simulink model "model_main5"  (R2023b)
settings: Solver=ode4  StartTime=0.0  StopTime=1000  FixedStep=dt  RelTol=1e-3
InitFcn:
  | model_init
values from neighbouring files (symbols this model uses):
  dt = 0.01    [model_init.m]
  Iws = diag([1 1 1 1])*0.2274    [model_init.m]
  m_tot = 3300    [model_init.m]
  norm_Ib = diag(diag(SC_Ib) / norm(diag(SC_Ib)))    [model_init.m]
  Omega1_init = 2000*rpm2rad    (= 209.439510239)    [model_init.m]
  Omega2_init = 2000*rpm2rad    (= 209.439510239)    [model_init.m]
  Omega3_init = 2000*rpm2rad    (= 209.439510239)    [model_init.m]
  Omega4_init = 2000*rpm2rad    (= 209.439510239)    [model_init.m]
  Omega_ref = [1000 1000 1000 1000]*rpm2rad    [model_init.m]
  port_offset = [7.196; 0 ; 0.618]    [model_init.m]
  qb0 = angle2quat(ag0(1),ag0(2),ag0(3),'ZYX')'    [model_init.m]
  rad2rpm = 1/rpm2rad    (= 9.54929658551)    [model_init.m]
  RCS_F = 1.0    (= 1)    [model_init.m]
  RCS_Pos = [RCS1_POS , RCS2_POS , RCS3_POS , RCS4_POS ,            RCS5_POS , RCS6_POS , RCS7_POS , RCS8_POS ,            RCS9_POS , RCS10_POS, RCS11_POS, RCS12_POS,            RCS13_POS, RCS14_POS, RCS15_POS, RCS16_POS]    [model_init.m]
  RCS_PWM_Freq = 0.1    [model_init.m]
  RCS_Sampling_time = 0.01    [model_init.m]
  RCS_THR_vec = [RCS1_THR , RCS2_THR , RCS3_THR , RCS4_THR,                 RCS5_THR , RCS6_THR , RCS7_THR , RCS8_THR,                 RCS9_THR , RCS10_THR, RCS11_THR, RCS12_THR,                 RCS13_THR, RCS14_THR, RCS15_THR, RCS16_THR]    [model_init.m]
  REL_port_POS_I_0 = REL_TS_POS_I_0 - quat2rotm(qb0') * port_offset    [model_init.m]
  REL_port_VEL_I_0 = REL_TS_VEL_I_0 - quat2rotm(qb0') * cross(wb0,port_offset)    [model_init.m]
  REL_TS_POS_I_0 = TS_pos0 - SC_pos0    [model_init.m]
  REL_TS_VEL_I_0 = TS_vel0 - SC_vel0    [model_init.m]
  RW_As = [RW1_Axis,RW2_Axis,RW3_Axis,RW4_Axis]    [model_init.m]
  RW_Max_Speed = 4200*rpm2rad    (= 439.822971503)    [model_init.m]
  RW_t_max = 0.5    [model_init.m]
  SC_Ib = [1843.56  -0.0019  -803.89 ... (first row only)    [model_init.m]
  SC_state0 = kepel_statvec (SC_Kepler)    [model_init.m]
  TS_Ib = diag([1 1 1])    [model_init.m]
  TS_qb0 = angle2quat(deg2rad(0),deg2rad(0),deg2rad(0),'ZYX')'    [model_init.m]
  TS_state0 = kepel_statvec (TS_Kepler)    [model_init.m]
  TS_wb0 = deg2rad([0 0 0]')    [model_init.m]
  wb0 = deg2rad([-0.3 -0.1 0.2])'    [model_init.m]
undefined symbols (not defined in the file or in its folder): RCS_F_vec, RCS_pos, SS_Total_Mass, TC_Kepler
libraries: simulink x16, simulink_extras x16, aerolibutil x9, sharedtransform x8
(part 3 of 3)

== matlab function model_main5/Enabled Subsystem/QP Controller2 ==
  settings: updateMethod=DISCRETE
  data: RCS_F_cmd output; RCS_tau_cmd output; F_pd_in input; tau_pd_in input; u_rw_cmd output; tau_rw_body output; tau_dump_ref output; Omega_rw_in input; Omega_ref_in input; RW_max_speed input; F_rcs_max_in input; tau_rcs_max_in input; k_dump input; eta_rw input; eta_tau_rcs input; eta_F input; v_tau input; v_dump input; v_F input; dt input; s_tau output; s_dump output; s_F output; exitflag_out output
function [RCS_F_cmd, RCS_tau_cmd, u_rw_cmd, tau_rw_body, tau_dump_ref, s_tau, s_dump, s_F, exitflag_out] = ...
    QP_CA_RW_RCS_WRENCH(F_pd_in, tau_pd_in, Omega_rw_in, Omega_ref_in, ...
    RW_max_speed, F_rcs_max_in, tau_rcs_max_in, ...
    k_dump, eta_rw, eta_tau_rcs, eta_F,  v_tau, v_dump, v_F, dt)

% Wrench-level QP control allocation
% - RW  : actuator-level (4 wheel torques)
% - RCS : wrench-level (3-axis force + 3-axis torque)
%
% Decision variable:
% z = [u_rw(4); tau_rcs(3); F_rcs(3); s_tau(3); s_dump(3); s_F(3)] -> 19
%
% Equality constraints:
%   -As*u_rw + tau_rcs - s_tau   = tau_pd
%    tau_rcs       - s_dump      = tau_dump_ref
%    F_rcs         - s_F         = F_pd
%
% Inputs
%   F_pd_in        [3x1] desired body force from position PD [N]
%   tau_pd_in      [3x1] desired body torque from attitude PD [N*m]
%   Omega_rw_in    [4x1] current wheel speeds [rad/s]
%   Omega_ref_in   [4x1] desired wheel speeds [rad/s]
%   RW_max_speed   [1x1] wheel speed limit [rad/s]
%   F_rcs_max_in   [3x1] approximate RCS body force bounds [N]
%   tau_rcs_max_in [3x1] approximate RCS body torque bounds [N*m]
%   k_dump         [1x1] momentum dumping gain [1/s]
%   eta_rw         [1x1] RW effort weight
%   eta_F          [1x1] RCS force effort weight
%   eta_rcs        [1x1] RCS torque effort weight
%   v_tau          [1x1] attitude slack weight
%   v_dump         [1x1] dumping slack weight
%   v_F            [1x1] force slack weight
%   dt             [1x1] sample time [s]
%
% Outputs
%   RCS_F_cmd      [3x1] body force command to existing RCS allocator [N]
%   RCS_tau_cmd    [3x1] body torque command to existing RCS allocator [N*m]
%   u_rw_cmd       [4x1] wheel torque command [N*m]
%   tau_rw_body    [3x1] RW-generated body torque [N*m]
%   tau_dump_ref   [3x1] desired dumping torque reference [N*m]
%   s_tau          [3x1] attitude torque slack
%   s_dump         [3x1] dumping torque slack
%   s_F            [3x1] force slack
%   exitflag_out   [1x1] quadprog exitflag

persistent z_save

if isempty(z_save)
    z_save = zeros(19,1);
end

%% outputs
RCS_F_cmd    = zeros(3,1);
RCS_tau_cmd  = zeros(3,1);
u_rw_cmd     = zeros(4,1);
tau_rw_body  = zeros(3,1);
tau_dump_ref = zeros(3,1);
s_tau        = zeros(3,1);
s_dump       = zeros(3,1);
s_F          = zeros(3,1);
exitflag_out = 0;

% for i = 1:3
%     if F_pd_in(i) >= F_rcs_max_in(i)
%         F_pd_in(i) = F_rcs_max_in(i);
%     elseif F_pd_in(i) <= -F_rcs_max_in(i)
%         F_pd_in(i) = -F_rcs_max_in(i);
%     end
% end
% 

%% fixed-size local copies
F_pd = zeros(3,1);
F_pd(1) = F_pd_in(1);
F_pd(2) = F_pd_in(2);
F_pd(3) = F_pd_in(3);

tau_pd = zeros(3,1);
tau_pd(1) = tau_pd_in(1);
tau_pd(2) = tau_pd_in(2);
tau_pd(3) = tau_pd_in(3);

Omega_rw = zeros(4,1);
Omega_rw(1) = Omega_rw_in(1);
Omega_rw(2) = Omega_rw_in(2);
Omega_rw(3) = Omega_rw_in(3);
Omega_rw(4) = Omega_rw_in(4);

Omega_ref = zeros(4,1);
Omega_ref(1) = Omega_ref_in(1);
Omega_ref(2) = Omega_ref_in(2);
Omega_ref(3) = Omega_ref_in(3);
Omega_ref(4) = Omega_ref_in(4);

F_rcs_max = zeros(3,1);
F_rcs_max(1) = abs(F_rcs_max_in(1));
F_rcs_max(2) = abs(F_rcs_max_in(2));
F_rcs_max(3) = abs(F_rcs_max_in(3));

tau_rcs_max = zeros(3,1);
tau_rcs_max(1) = abs(tau_rcs_max_in(1));
tau_rcs_max(2) = abs(tau_rcs_max_in(2));
tau_rcs_max(3) = abs(tau_rcs_max_in(3));

if dt <= 1e-6
    dt = 1e-6;
end

if RW_max_speed <= 1e-6
    RW_max_speed = 1e-6;
end

%% RW geometry
% tau_rw_body = -As * u_rw
As = [ 0.70710678,  0.0,        -0.70710678,  0.0;
    0.0,         0.70710678,  0.0,        -0.70710678;
    0.70710678,  0.70710678,  0.70710678,  0.70710678 ];

% wheel spin inertias [kg*m^2]
Jw = 0.2274 * ones(4,1);

%% actuator limits
% RW torque limits
u_rw_max = 0.5 * ones(4,1)  ;
u_rw_min = -u_rw_max;

% RW torque-rate limits
du_max = 20.0 * ones(4,1);   % [N*m/s]
du_min = -du_max;

% RW speed limits
Omega_max = RW_max_speed * ones(4,1) - 10;
Omega_min = -Omega_max;

%% previous solution
z_prev = z_save;
u_prev = z_prev(1:4);

%% virtual momentum dumping torque
% tau_dump_ref = -k_dump * h_rw_err
% h_rw_err = As * diag(Jw) * (Omega_rw - Omega_ref)
omega_err = Omega_rw - Omega_ref;
h_rw_err  = As * (Jw .* omega_err);   % [N*m*s]
tau_dump_ref = -k_dump * h_rw_err;    % [N*m]

%% QP cost
% z = [u_rw(4); tau_rcs(3); F_rcs(3); s_tau(3); s_dump(3); s_F(3)]
H = zeros(19,19);
f = zeros(19,1);

% effort weights
H = 2*diag([eta_rw*ones(4,1); ...
    eta_tau_rcs*ones(3,1); ...
    eta_F*ones(3,1); ...
    v_tau*ones(3,1); ...
    v_dump*ones(3,1); ...
    v_F*ones(3,1);]);
%%%%%%%%%%%%%
u_rw_scale   = u_rw_max;               % [N*m]
tau_scale    = tau_rcs_max(:);         % [N*m]
F_scale      = F_rcs_max(:);           % [N]

s_tau_scale  = tau_rcs_max(:) + abs(As)*u_rw_max;           % [N*m]
s_dump_scale = tau_rcs_max(:);           % [N*m]
s_F_scale    = F_rcs_max(:);             % [N]

scale_vec = [u_rw_scale;
             tau_scale; 
             F_scale;
             s_tau_scale;
             s_dump_scale;
             s_F_scale];

weight_vec = [eta_rw      * ones(4,1);
              eta_tau_rcs * ones(3,1);
              eta_F       * ones(3,1);
              v_tau       * ones(3,1);
              v_dump      * ones(3,1);
              v_F         * ones(3,1)];

H = 2 * diag(weight_vec ./ (scale_vec.^2  ));
%%%%%%%%%%%%%
% optional small RW smoothing
wr = 1e-3;
H(1,1) = H(1,1) + 2*wr;
H(2,2) = H(2,2) + 2*wr;
H(3,3) = H(3,3) + 2*wr;
H(4,4) = H(4,4) + 2*wr;
f(1:4) = -2*wr*u_prev;

% numerical symmetry
H = 0.5*(H + H') + 1e-9*eye(19);

%% equality constraints
% -As*u_rw + tau_rcs - s_tau  = tau_pd
%  tau_rcs       - s_dump     = tau_dump_ref
%  F_rcs         - s_F        = F_pd

Aeq = [       -As, eye(3), zeros(3,3),    -eye(3), zeros(3,3), zeros(3,3);
    zeros(3,4), eye(3), zeros(3,3), zeros(3,3),    -eye(3), zeros(3,3);
    zeros(3,4), zeros(3,3), eye(3), zeros(3,3), zeros(3,3),   -eye(3)];

beq = [tau_pd;
    tau_dump_ref;
    F_pd];

%% bounds
% RW torque-rate bounds
lb_rate = u_prev + du_min * dt;
ub_rate = u_prev + du_max * dt;

% RW speed-next bounds
% Omega_next = Omega_rw + dt*(u_rw./Jw)
lb_speed = Jw .* ((Omega_min - Omega_rw) / dt);
ub_speed = Jw .* ((Omega_max - Omega_rw) / dt);

% final RW bounds
lb_u = max(u_rw_min, max(lb_rate, lb_speed));
ub_u = min(u_rw_max, min(ub_rate, ub_speed));


% feasibility repair
for i = 1:4
    if lb_u(i) > ub_u(i)
        c = 0.5 * (lb_u(i) + ub_u(i));
        lb_u(i) = c;
        ub_u(i) = c;
    end
end

% RCS force bounds
lb_F = -F_rcs_max;
ub_F =  F_rcs_max;

% RCS torque bounds
lb_t = -tau_rcs_max;
ub_t =  tau_rcs_max;

% slack bounds
big = 1e6;
lb_s_tau  = -big * ones(3,1);
ub_s_tau  =  big * ones(3,1);
lb_s_dump = -big * ones(3,1);
ub_s_dump =  big * ones(3,1);
lb_s_F    = -big * ones(3,1);
ub_s_F    =  big * ones(3,1);

lb = [lb_u; lb_t; lb_F; lb_s_tau; lb_s_dump; lb_s_F];
ub = [ub_u; ub_t; ub_F; ub_s_tau; ub_s_dump; ub_s_F];

%% initial guess (make it equality-feasible)
u0 = min(max(u_prev, lb_u), ub_u);

F0 = F_pd;
for i = 1:3
    if F0(i) > ub_F(i)
        F0(i) = ub_F(i);
    elseif F0(i) < lb_F(i)
        F0(i) = lb_F(i);
    end
end

t0 = tau_dump_ref;
for i = 1:3
    if t0(i) > ub_t(i)
        t0(i) = ub_t(i);
    elseif t0(i) < lb_t(i)
        t0(i) = lb_t(i);
    end
end

s_tau0  = -As*u0 + t0 - tau_pd;
s_dump0 = t0 - tau_dump_ref;
s_F0    = F0 - F_pd;

x0 = [u0;
    t0;
    F0;
    s_tau0;
    s_dump0;
    s_F0];

%% solve
A = zeros(0,19);
b = zeros(0,1);

options = optimoptions('quadprog', ...
    'Algorithm', 'active-set', ...
    'Display', 'off', ...
    'ConstraintTolerance', 1e-6, ...
    'OptimalityTolerance', 1e-6, ...
    'StepTolerance', 1e-12, ...
    'MaxIterations', 60);

[z, ~, exitflag] = quadprog(H, f, A, b, Aeq, beq, lb, ub, x0, options);

if isempty(z) || exitflag <= 0
    z = x0;
end

%% outputs
u_rw_cmd    = z(1:4);
RCS_tau_cmd = z(5:7);
RCS_F_cmd   = z(8:10);

s_tau  = z(11:13);
s_dump = z(14:16);
s_F    = z(17:19);

tau_rw_body = -As * u_rw_cmd;

z_save = z;
exitflag_out = exitflag;
end

== matlab function model_main5/probe1 ==
  data: TS_p_I input; rel_port_pos output; SS_p_I input; TS_v_I input; SS_v_I input; q input; wb input; port_offset input; rel_port_vel output
function [rel_port_pos, rel_port_vel] = fcn(TS_p_I, SS_p_I, TS_v_I, SS_v_I, q, wb, port_offset) 
% port_offset : chaser CG-docking port offset    [7.196; 0 ; 0.618]
% q : body to eci
 
 
port_pos_I = SS_p_I + quat_to_dcm_sf(q) * port_offset;
port_vel_I = SS_v_I + quat_to_dcm_sf(q) * cross(wb,port_offset);

% Relative position based on docking ports

rel_port_pos = TS_p_I - port_pos_I;
rel_port_vel = TS_v_I - port_vel_I;
 
end

function C = quat_to_dcm_sf(q)
% scalar-first quaternion, body -> reference   quat2rotm
q = q / (sqrt(sum(q.^2)) + 1e-12);

qw = q(1);
qx = q(2);
qy = q(3);
qz = q(4);

C = [1-2*(qy*qy+qz*qz),   2*(qx*qy-qw*qz),   2*(qx*qz+qw*qy);
    2*(qx*qy+qw*qz),     1-2*(qx*qx+qz*qz), 2*(qy*qz-qw*qx);
    2*(qx*qz-qw*qy),     2*(qy*qz+qw*qx),   1-2*(qx*qx+qy*qy)];
end

== matlab function model_main5/Enabled Subsystem/QP Controller1 ==
  settings: updateMethod=DISCRETE
  data: RCS_F_cmd output; RCS_tau_cmd output; F_pd_in input; tau_pd_in input; u_rw_cmd output; Omega_rw_in input; Omega_ref_in input; RW_max_speed input; tau_rcs_max_in input; k_dump input; eta_rw input; eta_rcs input; v1 input; v2 input; dt input; tau_F_cmd output; tau_rw_body output; tau_dump_ref output; s1 output; s2 output; exitflag_out output
function [RCS_F_cmd, RCS_tau_cmd, u_rw_cmd, tau_F_cmd, tau_rw_body, tau_dump_ref, s1, s2, exitflag_out] = ...
    QP_CA_RW_RCS3(F_pd_in, tau_pd_in, Omega_rw_in, Omega_ref_in, ...
                  RW_max_speed, tau_rcs_max_in, ...
                  k_dump, eta_rw, eta_rcs, v1, v2, dt)
%#codegen
%
% QP control allocation based on the structure of Sec. 3.1,
% simplified to:
%   - RW (internal actuator)
%   - lumped 3-axis external torque command (for later RCS allocation)
%
% Decision variable:
%   z = [u_rw(4); tau_rcs(3); s1(3); s2(3)]  -> 13 states
%
% Equality constraints:
%   -As*u_rw + tau_rcs - s1 = tau_pd
%    tau_rcs - s2           = tau_dump_ref
%
% Inputs
%   tau_pd_in      [3x1] desired attitude body torque from high-level controller [N*m]
%   Omega_rw_in    [4x1] current RW speeds [rad/s]
%   Omega_ref_in   [4x1] desired RW speed reference [rad/s]
%   RW_max_speed   [1x1] RW speed limit [rad/s]
%   tau_rcs_max_in [3x1] max body torque envelope available from RCS [N*m]
%   k_dump         [1x1] momentum dumping gain [1/s]
%   eta_rw         [1x1] RW effort weight
%   eta_rcs        [1x1] external torque effort weight
%   v1             [1x1] attitude slack weight
%   v2             [1x1] dumping slack weight
%   dt             [1x1] sample time [s]
%
% Outputs
%   u_rw_cmd       [4x1] RW motor torque command [N*m]
%   tau_rcs_cmd    [3x1] desired 3-axis body torque for RCS allocation [N*m]
%   tau_rw_body    [3x1] body torque generated by RW [N*m]
%   tau_dump_ref   [3x1] desired external dumping torque [N*m]
%   s1             [3x1] attitude torque slack
%   s2             [3x1] dumping torque slack
%   exitflag_out   [1x1] quadprog exitflag

persistent z_save;

if isempty(z_save)
    z_save = zeros(13,1);
end

%% outputs
u_rw_cmd     = zeros(4,1);
RCS_tau_cmd  = zeros(3,1);
tau_rw_body  = zeros(3,1);
tau_dump_ref = zeros(3,1);
s1           = zeros(3,1);
s2           = zeros(3,1);
exitflag_out = 0;

%% fixed-size local copies
tau_pd = zeros(3,1);
tau_pd(1) = tau_pd_in(1);
tau_pd(2) = tau_pd_in(2);
tau_pd(3) = tau_pd_in(3);

Omega_rw = zeros(4,1);
Omega_rw(1) = Omega_rw_in(1);
Omega_rw(2) = Omega_rw_in(2);
Omega_rw(3) = Omega_rw_in(3);
Omega_rw(4) = Omega_rw_in(4);

Omega_ref = zeros(4,1);
Omega_ref(1) = Omega_ref_in(1);
Omega_ref(2) = Omega_ref_in(2);
Omega_ref(3) = Omega_ref_in(3);
Omega_ref(4) = Omega_ref_in(4);

tau_rcs_max = zeros(3,1);
tau_rcs_max(1) = abs(tau_rcs_max_in(1));
tau_rcs_max(2) = abs(tau_rcs_max_in(2));
tau_rcs_max(3) = abs(tau_rcs_max_in(3));

if dt <= 1e-6
    dt = 1e-6;
end

if RW_max_speed <= 1e-6
    RW_max_speed = 1e-6;
end

%% RW geometry
% tau_rw_body = -As * u_rw
As = [ 0.70710678,  0.0,        -0.70710678,  0.0;
       0.0,         0.70710678,  0.0,        -0.70710678;
       0.70710678,  0.70710678,  0.70710678,  0.70710678 ];

% wheel spin inertias [kg*m^2]
Jw = 0.227 * ones(4,1);

%% actuator limits
% RW torque limits
u_rw_max = 0.5 * ones(4,1);
u_rw_min = -u_rw_max;

% RW torque-rate limits
du_max = 2.0 * ones(4,1);   % [N*m/s]
du_min = -du_max;

% RW speed limits
Omega_max = RW_max_speed * ones(4,1);
Omega_min = -Omega_max;

%% previous solution
z_prev = z_save;
u_prev = z_prev(1:4);

%% virtual momentum dumping torque
% Paper uses u_h = -k_h * (...) * Cw*Jw*omega_w,e
% Here simplified for RCS-only external torque:
%   tau_dump_ref = -k_dump * h_rw_err
% where h_rw_err = As * diag(Jw) * (Omega_rw - Omega_ref)

omega_err = Omega_rw - Omega_ref;
h_rw_err  = As * (Jw .* omega_err);   % [N*m*s]
tau_dump_ref = -k_dump * h_rw_err;    % [N*m]

%% QP cost
% z = [u_rw(4); tau_rcs(3); s1(3); s2(3)]
H = zeros(13,13);
f = zeros(13,1);

% effort weights
H(1,1) = 2*eta_rw; H(2,2) = 2*eta_rw; H(3,3) = 2*eta_rw; H(4,4) = 2*eta_rw;
H(5,5) = 2*eta_rcs; H(6,6) = 2*eta_rcs; H(7,7) = 2*eta_rcs;
H(8,8) = 2*v1; H(9,9) = 2*v1; H(10,10) = 2*v1;
H(11,11) = 2*v2; H(12,12) = 2*v2; H(13,13) = 2*v2;

% optional small RW smoothing
wr = 1e-3;
H(1,1) = H(1,1) + 2*wr;
H(2,2) = H(2,2) + 2*wr;
H(3,3) = H(3,3) + 2*wr;
H(4,4) = H(4,4) + 2*wr;

f(1:4) = -2*wr*u_prev;

% numerical symmetry
H = 0.5*(H + H') + 1e-9*eye(13);

%% equality constraints
% -As*u_rw + tau_rcs - s1 = tau_pd
%  tau_rcs - s2           = tau_dump_ref

Aeq = [      -As, eye(3),    -eye(3), zeros(3,3);
       zeros(3,4), eye(3), zeros(3,3),   -eye(3)];

beq = [tau_pd;
       tau_dump_ref];

%% bounds
% RW torque-rate bounds
lb_rate = u_prev + du_min * dt;
ub_rate = u_prev + du_max * dt;

% RW speed-next bounds
% Omega_next = Omega_rw + dt*(u_rw./Jw)
lb_speed = Jw .* ((Omega_min - Omega_rw) / dt);
ub_speed = Jw .* ((Omega_max - Omega_rw) / dt);

% final RW bounds
lb_u = max(u_rw_min, max(lb_rate, lb_speed));
ub_u = min(u_rw_max, min(ub_rate, ub_speed));

% feasibility repair
for i = 1:4
    if lb_u(i) > ub_u(i)
        c = 0.5 * (lb_u(i) + ub_u(i));
        lb_u(i) = c;
        ub_u(i) = c;
    end
end

% external torque bounds
lb_t = -tau_rcs_max;
ub_t =  tau_rcs_max;

% slack bounds
big = 1e6;
lb_s1 = -big * ones(3,1);
ub_s1 =  big * ones(3,1);
lb_s2 = -big * ones(3,1);
ub_s2 =  big * ones(3,1);

lb = [lb_u; lb_t; lb_s1; lb_s2];
ub = [ub_u; ub_t; ub_s1; ub_s2];

%% initial guess (make it equality-feasible)
u0 = min(max(u_prev, lb_u), ub_u);

t0 = tau_dump_ref;
for i = 1:3
    if t0(i) > ub_t(i)
        t0(i) = ub_t(i);
    elseif t0(i) < lb_t(i)
        t0(i) = lb_t(i);
    end
end

s10 = -As*u0 + t0 - tau_pd;
s20 = t0 - tau_dump_ref;

x0 = [u0;
      t0;
      s10;
      s20];

%% solve
A = zeros(0,13);
b = zeros(0,1);

options = optimoptions('quadprog', ...
    'Algorithm', 'active-set', ...
    'Display', 'off', ...
    'ConstraintTolerance', 1e-6, ...
    'OptimalityTolerance', 1e-6, ...
    'StepTolerance', 1e-12, ...
    'MaxIterations', 50);

[z, ~, exitflag] = quadprog(H, f, A, b, Aeq, beq, lb, ub, x0, options);

if isempty(z) || exitflag <= 0
    z = x0;
end

%% outputs
u_rw_cmd    = z(1:4);
RCS_tau_cmd = z(5:7);
s1          = z(8:10);
s2          = z(11:13);

tau_rw_body = -As * u_rw_cmd;

z_save = z;
exitflag_out = exitflag;

end

== matlab function model_main5/Subsystem/QP_RCS_duty/QP Controller2 ==
  settings: updateMethod=DISCRETE
  data: RCS_duty_cmd output; RCS_F_est output; RCS_tau_est output; F_pd_in input; tau_pd_in input; u_rw_cmd output; tau_rw_body output; tau_dump_ref output; Omega_rw_in input; Omega_ref_in input; RW_max_speed input; RCS_pos_in input; RCS_thr_vec_in input; Tmax_in input; k_dump input; eta_rw input; eta_tau_rcs input; eta_F input; v_tau input; v_dump input; v_F input; dt input; s_tau output; s_dump output; s_F output; exitflag_out output
function [RCS_duty_cmd, RCS_F_est, RCS_tau_est, u_rw_cmd, tau_rw_body, ...
          tau_dump_ref, s_tau, s_dump, s_F, exitflag_out] = ...
    QP_CA_RW_RCS_DUTY(F_pd_in, tau_pd_in, Omega_rw_in, Omega_ref_in, ...
                      RW_max_speed, RCS_pos_in, RCS_thr_vec_in, Tmax_in, ...
                      k_dump, eta_rw, eta_tau_rcs, eta_F, ...
                      v_tau, v_dump, v_F, dt)
%#codegen
%
% Duty-level QP control allocation
%
% Decision variable:
% z = [u_rw(4); d_rcs(16); s_tau(3); s_dump(3); s_F(3)] -> 29
%
% Equality constraints:
%   -As*u_rw + Tmat*d_rcs - s_tau  = tau_pd
%             Tmat*d_rcs - s_dump  = tau_dump_ref
%             Fmat*d_rcs - s_F     = F_pd
%
% RCS exact actuator constraints:
%   0 <= d_rcs(i) <= 1

persistent z_save
 
if isempty(z_save)
    z_save = zeros(29,1);
end

%% outputs
RCS_duty_cmd = zeros(16,1);
RCS_F_est    = zeros(3,1);
RCS_tau_est  = zeros(3,1);
u_rw_cmd     = zeros(4,1);
tau_rw_body  = zeros(3,1);
tau_dump_ref = zeros(3,1);
s_tau        = zeros(3,1);
s_dump       = zeros(3,1);
s_F          = zeros(3,1);
exitflag_out = 0;

%% fixed-size local copies
F_pd = zeros(3,1);
F_pd(1) = F_pd_in(1);
F_pd(2) = F_pd_in(2);
F_pd(3) = F_pd_in(3);

tau_pd = zeros(3,1);
tau_pd(1) = tau_pd_in(1);
tau_pd(2) = tau_pd_in(2);
tau_pd(3) = tau_pd_in(3);

Omega_rw = zeros(4,1);
Omega_rw(1) = Omega_rw_in(1);
Omega_rw(2) = Omega_rw_in(2);
Omega_rw(3) = Omega_rw_in(3);
Omega_rw(4) = Omega_rw_in(4);

Omega_ref = zeros(4,1);
Omega_ref(1) = Omega_ref_in(1);
Omega_ref(2) = Omega_ref_in(2);
Omega_ref(3) = Omega_ref_in(3);
Omega_ref(4) = Omega_ref_in(4);

RCS_pos = zeros(3,16);
RCS_thr = zeros(3,16);
for i = 1:16
    RCS_pos(1,i) = RCS_pos_in(1,i);
    RCS_pos(2,i) = RCS_pos_in(2,i);
    RCS_pos(3,i) = RCS_pos_in(3,i);

    RCS_thr(1,i) = RCS_thr_vec_in(1,i);
    RCS_thr(2,i) = RCS_thr_vec_in(2,i);
    RCS_thr(3,i) = RCS_thr_vec_in(3,i);
end

if dt <= 1e-6
    dt = 1e-6;
end

if RW_max_speed <= 1e-6
    RW_max_speed = 1e-6;
end

if Tmax_in <= 1e-9
    Tmax_in = 1e-9;
end

%% RW geometry
% tau_rw_body = -As * u_rw
As = [ 0.70710678,  0.0,        -0.70710678,  0.0;
       0.0,         0.70710678,  0.0,        -0.70710678;
       0.70710678,  0.70710678,  0.70710678,  0.70710678 ];

% wheel spin inertias [kg*m^2]
Jw = 0.2274 * ones(4,1);

%% build RCS force/torque effectiveness matrices
Fmat = zeros(3,16);
Tmat = zeros(3,16);

for i = 1:16
    dir_i = RCS_thr(:,i);
    nrm = sqrt(dir_i(1)^2 + dir_i(2)^2 + dir_i(3)^2);
    if nrm > 1e-12
        dir_i = dir_i / nrm;
    else
        dir_i = [0;0;0];
    end

    Fi = Tmax_in * dir_i;
    Ti = cross3(RCS_pos(:,i), Fi);

    Fmat(:,i) = Fi;
    Tmat(:,i) = Ti;
end

%% actuator limits
% RW torque limits
u_rw_max = 0.5 * ones(4,1);
u_rw_min = -u_rw_max;

% RW torque-rate limits
du_max = 20.0 * ones(4,1);   % [N*m/s]
du_min = -du_max;

% RW speed limits
Omega_max = RW_max_speed * ones(4,1);
Omega_min = -Omega_max;

% RCS duty limits
d_min = zeros(16,1);
d_max = ones(16,1);

%% previous solution
z_prev = z_save;
u_prev = z_prev(1:4);
d_prev = z_prev(5:20);

%% momentum dumping reference
omega_err = Omega_rw - Omega_ref;
h_rw_err  = As * (Jw .* omega_err);   % [N*m*s]
tau_dump_ref = -k_dump * h_rw_err;    % [N*m]

%% QP cost
% z = [u_rw(4); d_rcs(16); s_tau(3); s_dump(3); s_F(3)]
H = zeros(29,29);
f = zeros(29,1);

% RW effort
H(1:4,1:4) = eta_rw * eye(4);

% RCS duty block
% torque/force magnitude penalty directly through achieved wrench
Hd = eta_tau_rcs * (Tmat' * Tmat) + eta_F * (Fmat' * Fmat);

% small regularization + duty smoothing
wd = 1e-4;
Hd = Hd + wd * eye(16);
H(5:20,5:20) = Hd;
f(5:20) = -wd * d_prev;

% RW smoothing
wr = 1e-3;
H(1:4,1:4) = H(1:4,1:4) + wr * eye(4);
f(1:4) = -wr * u_prev;

% slack weights
H(21:23,21:23) = v_tau  * eye(3);
H(24:26,24:26) = v_dump * eye(3);
H(27:29,27:29) = v_F    * eye(3);

% numerical symmetry
H = 0.5*(H + H') + 1e-9*eye(29);

%% equality constraints
% -As*u_rw + Tmat*d_rcs - s_tau  = tau_pd
%             Tmat*d_rcs - s_dump = tau_dump_ref
%             Fmat*d_rcs - s_F    = F_pd

Aeq = [      -As, Tmat, -eye(3), zeros(3,3), zeros(3,3);
       zeros(3,4), Tmat, zeros(3,3), -eye(3), zeros(3,3);
       zeros(3,4), Fmat, zeros(3,3), zeros(3,3), -eye(3)];

beq = [tau_pd;
       tau_dump_ref;
       F_pd];

%% bounds
% RW torque-rate bounds
lb_rate = u_prev + du_min * dt;
ub_rate = u_prev + du_max * dt;

% RW speed-next bounds
lb_speed = Jw .* ((Omega_min - Omega_rw) / dt);
ub_speed = Jw .* ((Omega_max - Omega_rw) / dt);

% final RW bounds
lb_u = max(u_rw_min, max(lb_rate, lb_speed));
ub_u = min(u_rw_max, min(ub_rate, ub_speed));

% feasibility repair
for i = 1:4
    if lb_u(i) > ub_u(i)
        c = 0.5 * (lb_u(i) + ub_u(i));
        lb_u(i) = c;
        ub_u(i) = c;
    end
end

% slack bounds
big = 1e6;
lb_s_tau  = -big * ones(3,1);
ub_s_tau  =  big * ones(3,1);
lb_s_dump = -big * ones(3,1);
ub_s_dump =  big * ones(3,1);
lb_s_F    = -big * ones(3,1);
ub_s_F    =  big * ones(3,1);

lb = [lb_u; d_min; lb_s_tau; lb_s_dump; lb_s_F];
ub = [ub_u; d_max; ub_s_tau; ub_s_dump; ub_s_F];

%% initial guess (equality-feasible)
u0 = min(max(u_prev, lb_u), ub_u);
d0 = min(max(d_prev, d_min), d_max);

tau0 = Tmat * d0;
F0   = Fmat * d0;

s_tau0  = -As*u0 + tau0 - tau_pd;
s_dump0 = tau0 - tau_dump_ref;
s_F0    = F0 - F_pd;

x0 = [u0;
      d0;
      s_tau0;
      s_dump0;
      s_F0];

%% solve
A = zeros(0,29);
b = zeros(0,1);

options = optimoptions('quadprog', ...
    'Algorithm', 'active-set', ...
    'Display', 'off', ...
    'ConstraintTolerance', 1e-6, ...
    'OptimalityTolerance', 1e-6, ...
    'StepTolerance', 1e-12, ...
    'MaxIterations', 60);

[z, ~, exitflag] = quadprog(H, f, A, b, Aeq, beq, lb, ub, x0, options);

if isempty(z) || exitflag <= 0
    z = x0;
end

%% outputs
u_rw_cmd     = z(1:4);
RCS_duty_cmd = z(5:20);

s_tau  = z(21:23);
s_dump = z(24:26);
s_F    = z(27:29);

RCS_F_est   = Fmat * RCS_duty_cmd;
RCS_tau_est = Tmat * RCS_duty_cmd;
tau_rw_body = -As * u_rw_cmd;

z_save = z;
exitflag_out = exitflag;

end

function c = cross3(a, b)
c = [ a(2)*b(3) - a(3)*b(2);
      a(3)*b(1) - a(1)*b(3);
      a(1)*b(2) - a(2)*b(1) ];
end

== matlab function model_main5/Subsystem/Attitude_PD_control ==
  settings: updateMethod=DISCRETE
  data: u_torq output; q_err input; w_err input
function u_torq = att_pd_control(q_err, w_err)

persistent first_flg
persistent I_save

dt = 0.01;

if isempty(first_flg)
    first_flg = 1;
    I_save = [0 0 0]';
end

K1 = 10.1*diag([1 1 1]);
K2 = 8.2*diag([1 1 1]);
K3 = 0.1*diag([1 1 1]);

q_err_ = [q_err(2), q_err(3), q_err(4)]';

u_torq = K1*q_err_ + K2*w_err + K3*I_save;

I_save = I_save + q_err_ * dt;

end

== matlab function model_main5/Subsystem/THR_Allocation ==
  data: pwm output; tau_cmd input; F_on input; f input; r_thr input
function pwm = RCS_Torque2PWM(tau_cmd, F_on, f, r_thr)
%#codegen
% ============================================================
% Minimal RCS allocation: torque command -> PWM duty (0..1)
%   tau ≈ sum_i r_i x (f_i * F_on_i * pwm_i)
%
% Inputs:
%   tau_cmd [3x1]
%   F_on    scalar or [12x1]
%   f       [3x12]  (columns are unit vectors)
%   r_thr   [3x12]  (columns are position vectors wrt CoM)
%
% Output:
%   pwm     [12x1] duty in [0,1]
% ============================================================
N = 16;
% F_on -> 12x1
if isscalar(F_on)
    Fon = F_on * ones(N,1);
else
    Fon = F_on(:);
end

% Build effectiveness matrix B (3x12): tau = B * pwm
B = zeros(3,N);
for i = 1:N
    Fi = Fon(i);
    B(:,i) = cross3(r_thr(:,i), f(:,i) * Fi);  % torque from pwm=1
end

% Unconstrained least-squares solution (minimum-norm)
pwm = B' * ((B*B') \ tau_cmd);

% Clamp to [0,1]
for i=1:N
    if pwm(i) < 0, pwm(i) = 0; end
    if pwm(i) > 1, pwm(i) = 1; end
end

end

function c = cross3(a,b)
c = [ a(2)*b(3) - a(3)*b(2);
      a(3)*b(1) - a(1)*b(3);
      a(1)*b(2) - a(2)*b(1) ];
end

== matlab function model_main5/Quaternion_Kinematics ==
  data: q input; w input; qd output
function qd = fcn(q,w)

F_q = (1/2)*[0 -w(1) -w(2) -w(3);
       w(1) 0 w(3) -w(2);
       w(2) -w(3) 0 w(1);
       w(3) w(2) -w(1) 0];

qd = F_q*q;

end

== matlab function model_main5/PWPFM/Subsystem17/MinOnTime_Enforcer1 ==
  settings: updateMethod=DISCRETE
  data: relay_raw input; F_gated output; t input
function F_gated = fcn(relay_raw, t)
%#codegen
% 최소 ON 시간 강제기 (MIB 기반)
% t_min_on = 0.0700 s (70 ms)
persistent t_on_start was_on;
if isempty(was_on)
    was_on     = false;
    t_on_start = 0;
end
t_min_on = 0.0700;
if relay_raw == 1 && ~was_on
    t_on_start = t;
end
if relay_raw == 1
    F_gated = 1;
elseif was_on && (t - t_on_start) < t_min_on
    F_gated = 1;   % 아직 70ms 안 됐으면 강제 ON 유지
else
    F_gated = 0;
end
was_on = (F_gated == 1);

end

== matlab function model_main5/Enabled Subsystem/QP  ==
  settings: updateMethod=DISCRETE
  data: tau_des input; u_rw_cmd output; Omega_rw input; dt input; tau_body_cmd output; exitflag_out output; RW_max_speed input; Iws input; As input
function [u_rw_cmd, tau_body_cmd, exitflag_out] = RW4_QP_Controller(tau_des, Omega_rw, dt, RW_max_speed, Iws, As)
%#codegen
%
% 4-wheel Reaction Wheel QP controller
% tau_body = -A_rw * u_rw
%
% Inputs:
%   tau_des   [3x1] desired body torque
%   Omega_rw  [4x1] current wheel speeds [rad/s]
%   u_prev    [4x1] previous wheel torque command [N*m]
%   dt        scalar control period [s]
%
% Outputs:
%   u_rw_cmd     [4x1] wheel motor torque command
%   tau_body_cmd [3x1] actual body torque from RW
%   exitflag_out scalar

persistent u_save;

if isempty(u_save)
    u_save = [0 0 0 0]';
end

u_rw_cmd     = zeros(4,1);
tau_body_cmd = zeros(3,1);
exitflag_out = 0;

tau_des  = reshape(tau_des,  [3,1]);
Omega_rw = reshape(Omega_rw, [4,1]);
u_prev   = u_save;

% =========================
% RW axis matrix (3x4)
% =========================
A_rw = [ 0.70710678,  0.0,        -0.70710678,  0.0;
         0.0,         0.70710678,  0.0,        -0.70710678;
         0.70710678,  0.70710678,  0.70710678,  0.70710678 ];

% =========================
% User parameters
% =========================
% Torque tracking weight (body torque tracking)
Wtau = diag([10.0, 10.0, 10.0]);

% Wheel torque magnitude penalty
Wu = 1e-3 * eye(4);

% Wheel torque smoothing penalty
Wr = 1e-2 * eye(4);

% Optional wheel-speed centering penalty
% Start with very small values. Increase later if wheel speeds drift too much.
Wh = zeros(4,4);
% 예: Wh = 1e-6 * eye(4);

% Wheel inertia about spin axis [kg*m^2]
Jw = 0.227*[1;1;1;1];

% Wheel torque limits [N*m]
u_max = [0.2; 0.2; 0.2; 0.2];
u_min = -u_max;

% Wheel torque rate limits [N*m/s]
du_max = [0.20; 0.20; 0.20; 0.20];
du_min = -du_max;

% Wheel speed limits [rad/s]
Omega_max = [RW_max_speed;RW_max_speed;RW_max_speed;RW_max_speed];
Omega_min = -Omega_max;

% =========================
% QP construction
%
% minimize 0.5*|| -A_rw*u - tau_des ||^2_Wtau
%        + 0.5*u'*Wu*u
%        + 0.5*(u-u_prev)'*Wr*(u-u_prev)
%        + 0.5*(Omega_next)'*Wh*(Omega_next)
%
% Omega_next = Omega_rw + D*u
% D = diag(dt./Jw)
% =========================

D = diag(dt ./ Jw);

H = A_rw' * Wtau * A_rw + Wu + Wr + D' * Wh * D;
f = A_rw' * Wtau * tau_des - Wr * u_prev + D' * Wh * Omega_rw;

% Make H numerically symmetric
H = 0.5 * (H + H');

% =========================
% Constraints
% 1) wheel torque bounds
% 2) wheel torque rate bounds
% 3) next-step wheel speed bounds
% =========================

% Torque-rate bounds
lb_rate = u_prev + du_min * dt;
ub_rate = u_prev + du_max * dt;

% Speed-next bounds
% Omega_next = Omega_rw + dt*(u./Jw)
% => u >= Jw .* (Omega_min - Omega_rw)/dt
% => u <= Jw .* (Omega_max - Omega_rw)/dt
lb_speed = Jw .* ((Omega_min - Omega_rw) / dt);
ub_speed = Jw .* ((Omega_max - Omega_rw) / dt);

% Final bounds
lb = max(u_min, max(lb_rate, lb_speed));
ub = min(u_max, min(ub_rate, ub_speed));

% Feasibility repair
for i = 1:4
    if lb(i) > ub(i)
        c = 0.5 * (lb(i) + ub(i));
        lb(i) = c;
        ub(i) = c;
    end
end

% Empty linear inequality/equality constraints
A   = zeros(0,4);
b   = zeros(0,1);
Aeq = zeros(0,4);
beq = zeros(0,1);

% Initial guess for active-set
x0 = min(max(u_prev, lb), ub);

% quadprog codegen-friendly option
options = optimoptions('quadprog', ...
    'Algorithm', 'active-set', ...
    'ConstraintTolerance', 1e-6, ...
    'OptimalityTolerance', 1e-6, ...
    'StepTolerance', 1e-12, ...
    'MaxIterations', 50);

[u_sol, ~, exitflag] = quadprog(H, f, A, b, Aeq, beq, lb, ub, x0, options);

if exitflag <= 0 || isempty(u_sol)
    u_rw_cmd = x0;
else
    u_rw_cmd = u_sol;
end

tau_body_cmd = -A_rw * u_rw_cmd;
u_save = u_rw_cmd;
exitflag_out = exitflag;

== matlab function model_main5/Subsystem/Get LOS Quaternion7 ==
  settings: updateMethod=DISCRETE
  data: r_rel input; v_rel input; r_ref input; v_ref input; a_ref input; q input; q_err input; w_err input; F_cmd_B output; tau_cmd_B output; m_sc input; Kp_pos input; Kd_pos input; Kp_att input; Kd_att input; r_err output; v_err output; q output; q_err_vec output; w_err output; a_cmd output
function [F_cmd_B, tau_cmd_B, r_err, v_err, q, q_err_vec, w_err, a_cmd] = ...
    relative_position_los_controller( ...
    r_rel, v_rel, ...          % [3x1] relative position/velocity
    r_ref, v_ref, a_ref, ...   % [3x1] desired relative pos/vel/acc
    q, q_err, w_err, ...                  % [4x1], [3x1] current attitude/angular velocity
    m_sc, Kp_pos, Kd_pos, Kp_att, Kd_att)
%#codegen
%
% q, q_los_ref : scalar-first quaternion [qw qx qy qz]'
%                body -> reference
% r_rel, r_ref, v_rel, v_ref, a_ref : reference frame 기준
%
% 출력:
% F_cmd_B   : [3x1] body frame force command
% tau_cmd_B : [3x1] body frame torque command

    F_cmd_B   = zeros(3,1);
    tau_cmd_B = zeros(3,1);
    r_err     = zeros(3,1);
    v_err     = zeros(3,1);
    q_err_vec = zeros(3,1);
    % w_err     = zeros(3,1);
    a_cmd     = zeros(3,1);

    %% 1) Relative position controller
    r_err = r_ref - r_rel;
    v_err = v_ref - v_rel;

    a_cmd = a_ref + Kp_pos * r_err + Kd_pos * v_err;
    F_cmd_R = m_sc * a_cmd;

    %% 2) Reference frame -> body frame
    % q : body -> reference
    % therefore F_B = C_BR' * F_R
    C_BR   = quat_to_dcm_sf(q);
    F_cmd_B = C_BR' * F_cmd_R;

    %% 3) LOS attitude controller

    % shortest path
    if q_err(1) < 0
        q_err = -q_err;
    end

    q_err_vec = q_err(2:4);

    tau_cmd_B = Kp_att * q_err_vec + Kd_att * w_err;
end


function q_out = quat_mul_sf(a, b)
% scalar-first quaternion multiplication
    q_out = [ a(1)*b(1) - a(2)*b(2) - a(3)*b(3) - a(4)*b(4);
              a(1)*b(2) + a(2)*b(1) + a(3)*b(4) - a(4)*b(3);
              a(1)*b(3) - a(2)*b(4) + a(3)*b(1) + a(4)*b(2);
              a(1)*b(4) + a(2)*b(3) - a(3)*b(2) + a(4)*b(1) ];
end


function C = quat_to_dcm_sf(q)
% scalar-first quaternion, body -> reference
    q = q / (sqrt(sum(q.^2)) + 1e-12);

    qw = q(1);
    qx = q(2);
    qy = q(3);
    qz = q(4);

    C = [1-2*(qy*qy+qz*qz),   2*(qx*qy-qw*qz),   2*(qx*qz+qw*qy);
         2*(qx*qy+qw*qz),     1-2*(qx*qx+qz*qz), 2*(qy*qz-qw*qx);
         2*(qx*qz-qw*qy),     2*(qy*qz+qw*qx),   1-2*(qx*qx+qy*qy)];
end

== matlab function model_main5/Subsystem/RCS_Relative_Position_Control_Allocation1 ==
  settings: updateMethod=DISCRETE
  data: F_cmd input; tau_cmd input; RCS_pos input; RCS_F_vec input; Tmax input; duty output; F_est output; tau_est output; F_err output; tau_err output; sat_ratio output; wF input; wT input
function [duty, F_est, tau_est, F_err, tau_err, sat_ratio] = ...
    rcs_force_torque_allocator(F_cmd, tau_cmd, RCS_pos, RCS_F_vec, Tmax, wF, wT)
%#codegen
%
% F_cmd      : [3x1] commanded force in body frame [N]
% tau_cmd    : [3x1] commanded torque in body frame [N*m]
% RCS_pos    : [3xN] thruster positions in body frame [m]
% RCS_F_vec  : [3xN] thruster direction vectors
% Tmax       : scalar, max thrust of one thruster [N]
% wF         : scalar, force tracking weight
% wT         : scalar, torque tracking weight
%
% duty       : [N x 1], 0~1
% F_est      : [3x1], achieved force [N]
% tau_est    : [3x1], achieved torque [N*m]
% F_err      : [3x1], force error [N]
% tau_err    : [3x1], torque error [N*m]
% sat_ratio  : saturated thruster ratio

    N = size(RCS_pos, 2);

    duty      = zeros(N,1);
    F_est     = zeros(3,1);
    tau_est   = zeros(3,1);
    F_err     = zeros(3,1);
    tau_err   = zeros(3,1);
    sat_ratio = 0;

    Fmat = zeros(3, N);
    Tmat = zeros(3, N);

    for i = 1:N
        dir_i = RCS_F_vec(:,i);
        nrm   = sqrt(sum(dir_i.^2));

        if nrm > 1e-12
            dir_i = dir_i / nrm;
        else
            dir_i = [0;0;0];
        end

        Fi = Tmax * dir_i;
        Ti = cross3(RCS_pos(:,i), Fi);

        Fmat(:,i) = Fi;
        Tmat(:,i) = Ti;
    end

    % Solve:
    % min || wF*(Fmat*u - F_cmd) ||^2 + || wT*(Tmat*u - tau_cmd) ||^2
    % s.t. 0 <= u <= 1

    A = [wF * Fmat;
         wT * Tmat];

    b = [wF * F_cmd;
         wT * tau_cmd];

    H = A' * A + 1e-8 * eye(N);
    g = A' * b;

    alpha = 1.0 / (trace(H) + 1e-9);
    u = zeros(N,1);

    for k = 1:150
        grad = H * u - g;
        u    = u - alpha * grad;

        for j = 1:N
            if u(j) < 0
                u(j) = 0;
            elseif u(j) > 1
                u(j) = 1;
            end
        end
    end

    duty    = u;
    F_est   = Fmat * duty;
    tau_est = Tmat * duty;

    F_err   = F_cmd   - F_est;
    tau_err = tau_cmd - tau_est;

    sat_ratio = sum(duty > 0.999) / N;
end


function c = cross3(a, b)
    c = [ a(2)*b(3) - a(3)*b(2);
          a(3)*b(1) - a(1)*b(3);
          a(1)*b(2) - a(2)*b(1) ];
end

== matlab function model_main5/Subsystem/SS Attitude Control wrt ECI ==
  settings: updateMethod=DISCRETE
  data: q_err input; RW_cmd output; w_err input; As input; Kp_rw input; Kd_rw input; Ki_rw input
function RW_cmd  = Att_PD_Control(q_err, w_err, As,Kp_rw,Kd_rw,Ki_rw)

persistent I_save
persistent flg

if isempty(flg)
    flg = 1;
    I_save = [0 0 0]';
end
 
% K3 = 0.025*diag([1 1 1]);

q_e_v = [q_err(2), q_err(3), q_err(4)]';

u = Kp_rw*q_e_v + Kd_rw*w_err + Ki_rw*I_save;

% RW_cmd = pinv(As)*-u;
RW_cmd = u; 

I_save = I_save + (q_e_v*0.01);

end

== matlab function model_main5/Subsystem/MATLAB Function1 ==
  data: kepel input; statvec output
function statvec  = kepel_statvec (kepel)
%  [statvec] = kepel_statvec (kepel)
%	The function kepel_statvec transforms the keplerian
%	elements kepel into the corresponding state vector in
%	the same reference system.
%
% Input:
%	kepel
% 		vector containing the keplerian elements:
%		(1) - semimajor axis of the orbit in meters.
%		(2) - eccentricity.
%		(3) - inclinatsion in radians.
%		(4) - right ascension of ascending node in radians.
%		(5) - argument of perigee in radians.
%		(6) - mean anomaly in radians.
% Output:
%	statvec
%  		state vector in meters and meters/second.
%
% Authors:
%	Helio K. Kuga;
%	Valder M. Medeiros;
%	Valdemir Carrara		february/80		version 1.0
%	Valdemir Carrara		july 2005		(C version)
%   Valdemir Carrara            March/09        Matlab

EARTH_GRAVITY	= 3.9860064e+14;		% Earth's gravitational constant (m**3/s**2)

a    = kepel(1);	% semi-major axis
exc  = kepel(2);	% eccentricity

c1   = sqrt(1. - exc*exc);

%     rotation matrix

orb2iner = rotmaz(-kepel(4))*rotmax(-kepel(3))*rotmaz(-kepel(5));

%     Kepler's equation

E    = kepler(kepel(6), exc);

sE   = sin(E);
cE   = cos(E);
c3   = sqrt(EARTH_GRAVITY/a)/(1. - exc*cE);

%     state vector

statvec = [[a*(cE - exc), a*c1*sE, 0]*orb2iner', [-c3*sE, c1*c3*cE, 0]*orb2iner'];

end

function [rot_mat] = rotmax (angle)
% [rot_mat] = rotmax (angle)
%   To obtain the rotation matrix around the X axis given the
%   rotation angle.
% inputs:
%   angle
%       rotation angle, in radians.
% outputs:
%   rot_mat
%       rotation matrix (3, 3)
%

% Valdemir Carrara, Sep, 1998

coan    =  cos(angle);
sian    =  sin(angle);

rot_mat =  [1, 0, 0; 0, coan, sian; 0, -sian, coan];

end

function [rot_mat] = rotmay (angle)
% [rot_mat] = rotmay (angle)
%   To obtain the rotation matrix around the Y axis given the
%   rotation angle.
% inputs:
%   angle
%       rotation angle, in radians.
% outputs:
%   rot_mat
%       rotation matrix (3, 3)
%

% Valdemir Carrara, Sep, 1998


coan    =  cos(angle);
sian    =  sin(angle);

rot_mat =  [coan, 0, -sian; 0, 1, 0; sian, 0, coan];

end

function [rot_mat] = rotmaz (angle)
% [rot_mat] = rotmaz (angle)
%   To obtain the rotation matrix around the Z axis given the
%   rotation angle.
% inputs:
%   angle
%       rotation angle, in radians.
% outputs:
%   rot_mat
%       rotation matrix (3, 3)
%

% Valdemir Carrara, Sep, 1998

coan    =  cos(angle);
sian    =  sin(angle);

rot_mat =  [coan, sian, 0; -sian, coan, 0; 0, 0, 1];
end

function [eccentric] = kepler (mean_anomaly, eccentricity)
% [eccentric] = kepler (mean_anomaly, eccentricity)
%	The subroutine kepler finds a solution to the
%	kepler's equation.
%
% Input:
%	mean_anomaly
%		mean anomaly in radians.
%	eccentricity
%		eccentricity.
%
% Output:
%	eccentric
%		eccentric anomaly in radians.
%
% Authors:
%	Valder M. de Medeiros		june/81		version 2.0
%	Valdemir Carrara			july 2005	(C version)
%   Valdemir Carrara            March/09        Matlab

exc2    = eccentricity*eccentricity;
am1     = mod (mean_anomaly, 2*pi);
am2     = am1 + am1;
am3     = am1 + am2;
shoot   = am1 + eccentricity*(1. - 0.125*exc2)*sin(am1) + ...
		0.5*exc2*(sin(am2) + 0.75*eccentricity*sin(am3));
shoot   = mod (shoot, 2*pi);

e1      = 1.0;
ic      = 0;

while ((abs(e1) > 1.e-12) && (ic <= 10)) 
	e1    = (shoot - am1 - eccentricity*sin(shoot)) / ...
			(1.0 - eccentricity*cos(shoot));
    shoot = shoot - e1;
    ic    = ic + 1;
end

if (ic >= 10)
    disp ('warning ** subroutine kepler did not converge in 10 iterations');
end

eccentric = shoot;


end

== matlab function model_main5/Subsystem/TC Kepler Propagate ==
  data: initial_condition input; dfdt output; F_eci input
function dfdt  = eq_propagate(initial_condition, F_eci)
% Lectures_TwoBodyProblem.pdf
% 우주시스템입문 - 도미타 노부유키 eq(7.8) p136
% https://en.wikipedia.org/wiki/Standard_gravitational_parameter
u  = 3.9860064e+14; % earth gravitional parameter
Re = 6378137;      % earth radius [m]

dfdt = zeros(size(initial_condition));

% x=x
% x1=dx/dt
% dx1/dt = d^2(x)/dt

x1 = initial_condition(4); % x1 = dx/dt
y1 = initial_condition(5); % y1 = dy/dt
z1 = initial_condition(6); % z1 = dz/dt
x  = initial_condition(1); % x
y  = initial_condition(2); % y
z  = initial_condition(3); % z

r=sqrt(x^2+y^2+z^2);

% % %   Keplar Motion Equatnion
% % %  => r_dd + u/(r^3)r_ = 0 => r_dd = -u/(r^3)r_
dfdt(1) = x1;
dfdt(2) = y1;
dfdt(3) = z1;
dfdt(4) = -u*x/(r^3) + F_eci(1);
dfdt(5) = -u*y/(r^3) + F_eci(2);
dfdt(6) = -u*z/(r^3) + F_eci(3);

end

== matlab function model_main5/SC 6-DOF Dynamics ==
  data: w input; x input; Ib input; m_tot input; Iws input; As input; Omega input; Omegad input; RCS_mea input; RCS_pos input; RCS_vec input; wd output; R_Ib input; T_ext input; F_ext input; xd output
function [wd, xd]  = eq_propagate(w, x, Ib, m_tot, ...
                                   Iws, As, Omega, Omegad, ...
                                   RCS_mea, RCS_pos, RCS_vec, R_Ib, ...
                                   T_ext, F_ext)
% % 
% 출력 1: 위성 동체 좌표계 각가속도
% 출력 2: 관성좌표계 선가속도

% % 
RW_h = As*Iws*Omega;
RW_hd = As*Iws*Omegad;

% % 
N = 16;
RCS_f = zeros(3,N);
RCS_t = zeros(3,N);

for i = 1:N
    r_i = RCS_pos(:,i);   % position of thruster i
    d_i = RCS_vec(:,i);   % thrust direction of thruster i

    % force contribution
    RCS_f(:,i) = d_i;

    % torque contribution
    RCS_t(:,i) = cross(r_i, d_i);
end
RCS_f_total = RCS_f * RCS_mea;  % [3x1]
RCS_t_total = RCS_t * RCS_mea;  % [3x1]


%% Rotational Motion
wd = [0 0 0]';
wd = inv(Ib)*(T_ext + RCS_t_total - RW_hd - cross(w, Ib*w + RW_h));

%% Translational Motion

F_I = R_Ib * RCS_f_total;

u  = 3.986004418e14; % earth gravitional parameter
Re = 6378137;        % earth radius [m]

xd = zeros(size(x));

v1_i = x(4); % x1 = dx/dt
v2_i = x(5); % y1 = dy/dt
v3_i = x(6); % z1 = dz/dt
p1_i = x(1); % x
p2_i = x(2); % y
p3_i = x(3); % z

r=sqrt(p1_i^2+p2_i^2+p3_i^2);

% % %   Keplar Motion Equatnion
% % %  => r_dd + u/(r^3)r_ = 0 => r_dd = -u/(r^3)r_
xd(1) = v1_i;
xd(2) = v2_i;
xd(3) = v3_i;
xd(4) = -u*p1_i/(r^3) + F_I(1)/m_tot + F_ext(1)/m_tot;
xd(5) = -u*p2_i/(r^3) + F_I(2)/m_tot + F_ext(2)/m_tot;
xd(6) = -u*p3_i/(r^3) + F_I(3)/m_tot + F_ext(3)/m_tot;

end

== matlab function model_main5/Quaternion_Kinematics1 ==
  data: q input; w input; qd output
function qd = fcn(q,w)

F_q = (1/2)*[0 -w(1) -w(2) -w(3);
       w(1) 0 w(3) -w(2);
       w(2) -w(3) 0 w(1);
       w(3) w(2) -w(1) 0];

qd = F_q*q;

end
